simulink model "Project_2"  (R2023a)
settings: Solver=VariableStepAuto  StartTime=0.0  StopTime=10.0  RelTol=1e-3
undefined symbols (not defined in the file): A, A1, A2, Cd, Cd1, Cd2, g, m, rho
settings Model: Creator=Aman  LastModifiedBy=Aman

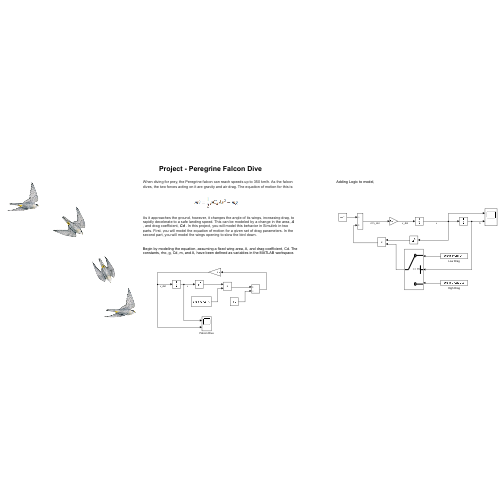
[thumbnail: Simulink's stored preview of the top-level diagram]
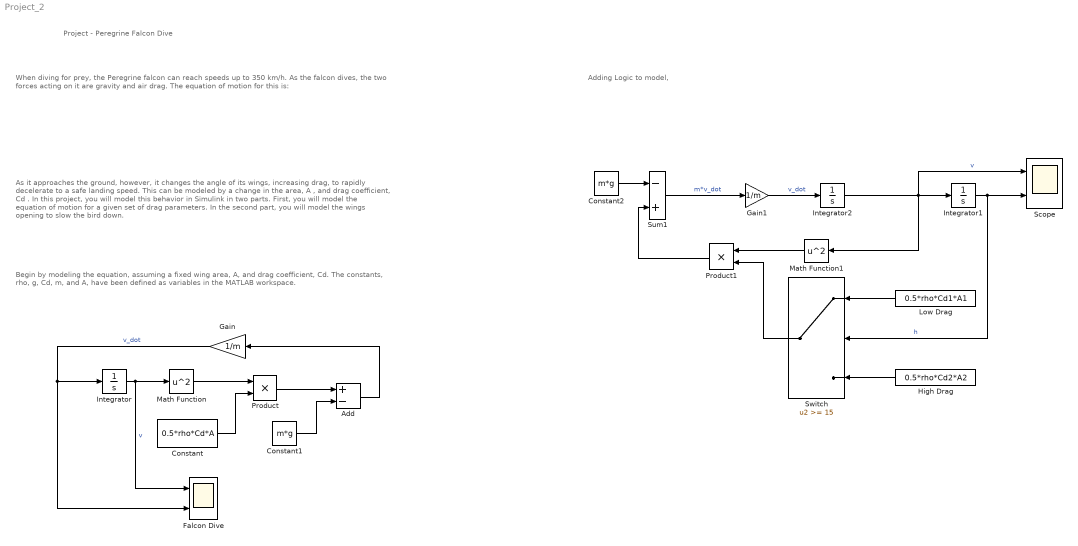
== system Project_2 ==
  note: Adding Logic to model,
  note: Begin by modeling the equation, assuming a fixed wing area, A, and drag coefficient, Cd. The constants, rho, g, Cd, m, and A, have been defined as variables in the MATLAB workspace.
  note: As it approaches the ground, however, it changes the angle of its wings, increasing drag, to rapidly decelerate to a safe landing speed. This can be modeled by a change in the area, A
      | , and drag coefficient, Cd . In this project, you will model this behavior in Simulink in two parts. First, you will model the equation of motion for a given set of drag parameters. In the second part, you will model the wings opening to slow the bird down.
  note: When diving for prey, the Peregrine falcon can reach speeds up to 350 km/h. As the falcon dives, the two forces acting on it are gravity and air drag. The equation of motion for this is:
  note: Project - Peregrine Falcon Dive
  Add : Sum  Inputs=+-
  Constant : Constant  Value=0.5*rho*Cd*A
  Constant1 : Constant  Value=m*g
  Constant2 : Constant  Value=m*g
  Falcon Dive : Scope  NumInputPorts=2
  Gain : Gain  Gain=1/m
  Gain1 : Gain  Gain=1/m
  High Drag : Constant  Value=0.5*rho*Cd2*A2
  Integrator : Integrator  InitialCondition=-10
  Integrator1 : Integrator  InitialCondition=60
  Integrator2 : Integrator  InitialCondition=-10
  Low Drag : Constant  Value=0.5*rho*Cd1*A1
  Math Function : Math  Operator=square
  Math Function1 : Math  Operator=square  SignedPower=on
  Product : Product
  Product1 : Product
  Scope : Scope  NumInputPorts=2
  Sum1 : Sum  Inputs=-+
  Switch : Switch  Threshold=15  SaturateOnIntegerOverflow=off  InputSameDT=off
  wires:
  Add/1 -> Gain/1
  Constant/1 -> Product/2
  Constant1/1 -> Add/2
  Product/1 -> Add/1
  Integrator/1 -> Falcon Dive/1, Math Function/1  "v"
  Gain/1 -> Integrator/1, Falcon Dive/2  "v_dot"
  Math Function/1 -> Product/1
  High Drag/1 -> Switch/3
  Low Drag/1 -> Switch/1
  Switch/1 -> Product1/2
  Gain1/1 -> Integrator2/1  "v_dot"
  Sum1/1 -> Gain1/1  "m*v_dot"
  Product1/1 -> Sum1/2
  Math Function1/1 -> Product1/1
  Integrator1/1 -> Scope/2, Switch/2  "h"
  Constant2/1 -> Sum1/1
  Integrator2/1 -> Scope/1, Math Function1/1, Integrator1/1  "v"
